simulink model "SkakacVRMLmodel"  (Simulink 7.7)
settings: Solver=ode45  StartTime=0.0  StopTime=inf  RelTol=1e-3
libraries: vrlib x1
settings Model: Creator=Alan Mutka  LastModifiedBy=Alan Mutka

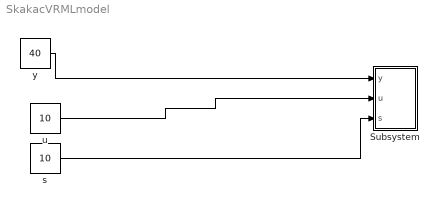
== system SkakacVRMLmodel ==
  Subsystem : Subsystem
  s : Constant  Value=10
  u : Constant  Value=10
  y : Constant  Value=40
  wires:
  u/1 -> Subsystem/2(u)
  y/1 -> Subsystem/1(y)
  s/1 -> Subsystem/3(s)

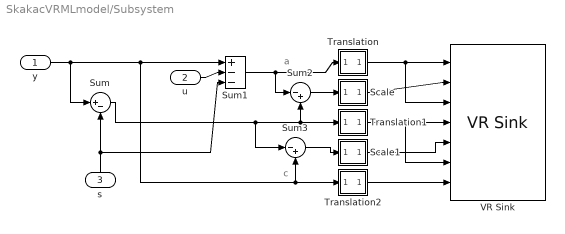
== system SkakacVRMLmodel/Subsystem ==
  note: a
  note: c
  y : Inport
  u : Inport  Port=2
  s : Inport  Port=3
  Scale : Subsystem
  Scale1 : Subsystem
  Sum : Sum  Inputs=|+-
  Sum1 : Sum  Inputs=|+--
  Sum2 : Sum  Inputs=|-+
  Sum3 : Sum  Inputs=|-+
  Translation : Subsystem
  Translation1 : Subsystem
  Translation2 : Subsystem
  VR Sink : vrlib/VR Sink  SampleTime=-1  ViewEnable=on  RemoteChange=off  RemoteView=on  FieldsWritten=ALFA.translation.3.1.1.double#Opruga.scale.3.1.1.double#Opruga.translation.3.1.1.double#MASS2.translation.3.1.1.double#PRISMATIC.scale.3.1.1.double#PRISMATIC.translation.3.1.1.double#MASS1.translation.3.1.1.double  WorldFileName=skakac2.WRL  AutoView=off  VideoDimensions=[]  FigureProperties="{'Position', 'Name', 'Viewpoint', 'CameraBound', 'CameraDirection', 'CameraPosition', 'CameraUpVector', 'ZoomFactor', 'Antialiasing', 'Headlight', 'Lighting', 'NavPanel', 'StatusBar', 'ToolBar', 'Textures', 'Transparency', 'Wireframe', 'NavZones', 'NavMode', 'NavSpeed', 'Record2DCompressMethod', 'Record2DCompressQuality', 'Record2D', 'Record2DFileName', 'Record2DFPS'; [5.0000000000000000e+000  9.2000000000000000e+001  5.7600000000000000e+002  3.8000000000000000e+002], '', '', 'on', [0.0000000000000000e+000  0.0000000000000000e+000 -1.0000000000000000e+000], [0.0000000000000000e+000  0.0000000000000000e+000  1.3200000000000000e+002], [0.0000000000000000e+000  1.0000000000000000e+000  0.0000000000000000e+000], [1.0000000000000000e+000], 'on', 'on', 'on', 'halfbar', 'on', 'on', 'on', 'on', 'off', 'off', 'fly', 'normal', 'auto', [7.5000000000000000e+001], 'off', '%f_anim_%n.avi', [1.5000000000000000e+001]}"
  wires:
  y/1 -> Sum3/2, Translation2/1(In1), Sum1/1, Sum/1
  s/1 -> Sum1/3, Sum/2
  Sum1/1 -> Translation/1(In1), Sum2/1
  Sum/1 -> Translation1/1(In1), Sum2/2, Sum3/1
  Translation/1(Out1) -> VR Sink/1, VR Sink/3
  Scale/1(Out1) -> VR Sink/2
  Translation1/1(Out1) -> VR Sink/4, VR Sink/6
  Translation2/1(Out1) -> VR Sink/7
  Sum2/1 -> Scale/1(In1)
  Sum3/1 -> Scale1/1(In1)
  Scale1/1(Out1) -> VR Sink/5
  u/1 -> Sum1/2

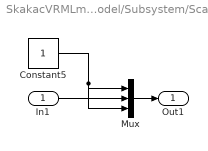
== system SkakacVRMLmodel/Subsystem/Scale ==
  In1 : Inport
  Constant5 : Constant
  Mux : Mux  Inputs=3
  Out1 : Outport
  wires:
  Mux/1 -> Out1/1
  In1/1 -> Mux/2
  Constant5/1 -> Mux/1, Mux/3

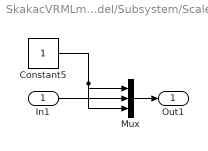
== system SkakacVRMLmodel/Subsystem/Scale1 ==
  In1 : Inport
  Constant5 : Constant
  Mux : Mux  Inputs=3
  Out1 : Outport
  wires:
  Constant5/1 -> Mux/3, Mux/1
  In1/1 -> Mux/2
  Mux/1 -> Out1/1

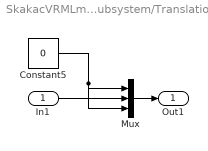
== system SkakacVRMLmodel/Subsystem/Translation ==
  In1 : Inport
  Constant5 : Constant  Value=0
  Mux : Mux  Inputs=3
  Out1 : Outport
  wires:
  Constant5/1 -> Mux/3, Mux/1
  In1/1 -> Mux/2
  Mux/1 -> Out1/1

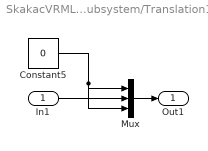
== system SkakacVRMLmodel/Subsystem/Translation1 ==
  In1 : Inport
  Constant5 : Constant  Value=0
  Mux : Mux  Inputs=3
  Out1 : Outport
  wires:
  Mux/1 -> Out1/1
  In1/1 -> Mux/2
  Constant5/1 -> Mux/1, Mux/3

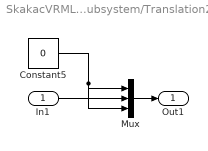
== system SkakacVRMLmodel/Subsystem/Translation2 ==
  In1 : Inport
  Constant5 : Constant  Value=0
  Mux : Mux  Inputs=3
  Out1 : Outport
  wires:
  Constant5/1 -> Mux/3, Mux/1
  In1/1 -> Mux/2
  Mux/1 -> Out1/1
